simulink model "full_controlled_rect"  (R2017a)
settings: Solver=FixedStepAuto  StartTime=0.0  StopTime=15  RelTol=1e-3  EnableMultiTasking=on
libraries: powerlib x9, powerlib_meascontrol x7
settings Model: Creator=Admin  LastModifiedBy=re
settings OptimizationCC: LifeSpan=inf
settings DebuggingCC: SFUnexpectedBacktrackingDiag=warning  SFNoUnconditionalDefaultTransitionDiag=warning  SFExecutionAtInitializationDiag=none
settings GRTTargetCC: TargetLangStandard=C89/C90 (ANSI)  GeneratePreprocessorConditionals=Disable all
settings ConfigComp: CovMetricSettings=dw  CovHtmlReporting=on  CovSaveCumulativeToWorkspaceVar=on  CovSaveSingleToWorkspaceVar=on  CovExternalEMLEnable=off

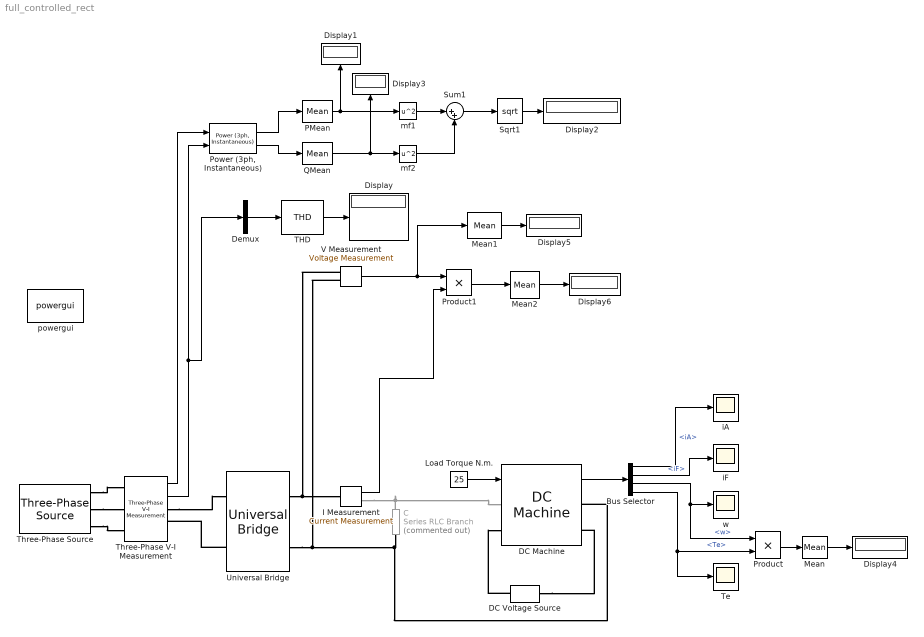
== system full_controlled_rect ==
  Bus Selector : BusSelector  OutputSignals=iA,iF,w,Te
  C : powerlib/Elements/Series RLC Branch  Commented=on  LConnTagsString=__new0  RConnTagsString=__new0  BranchType=RLC  Resistance=0  Inductance=0  SetiL0=off  InitialCurrent=0  Capacitance=100e-3  Setx0=off  InitialVoltage=0  Measurements=None
  DC Machine : powerlib/Machines/DC Machine  PresetModel=No  MechanicalLoad=Torque TL  FieldType=Wound  ShowDetailedParameters=on  MeasurementBus=on  RLa="[10  0.01]"  RLf="[300  156]"  Laf=2  MachineConstant=Torque constant (N.m/A)  Ke=1.8  Kt=1.8  J=1  Bm=0  Tf=0  w0=1  Ifinit=1  TsPowergui=0  TsBlock=-1
  DC Voltage Source : powerlib/Electrical Sources/DC Voltage Source  Amplitude=300  Measurements=None
  Demux : Demux  Outputs=1
  Display{,1..6} (7 alike) : Display
  I Measurement : powerlib/Measurements/Current Measurement  PhasorSimulation=off  OutputType=Complex  PSBequivalent=0
  Load Torque N.m. : Constant  Value=25
  Mean : powerlib_meascontrol/Measurements/Mean  Freq=60  Vinit=0  Ts=0
  Mean1 : powerlib_meascontrol/Measurements/Mean  Freq=60  Vinit=0  Ts=0
  Mean2 : powerlib_meascontrol/Measurements/Mean  Freq=60  Vinit=0  Ts=0
  PMean : powerlib_meascontrol/Measurements/Mean  Freq=60  Vinit=0  Ts=0
  "Power (3ph, Instantaneous)" : powerlib_meascontrol/Measurements/Power (3ph, Instantaneous)
      settings: SourceProductName=Simscape Power Systems
  Product : Product
  Product1 : Product
  QMean : powerlib_meascontrol/Measurements/Mean  Freq=60  Vinit=0  Ts=0
  Sqrt1 : Sqrt  SaturateOnIntegerOverflow=on
  Sum1 : Sum  Inputs=|++
  THD : powerlib_meascontrol/Measurements/THD  Freq=50  Ts=0
  Te : Scope
  Three-Phase V-I Measurement : powerlib/Measurements/Three-Phase V-I Measurement  VoltageMeasurement=phase-to-ground  SetLabelV=off  LabelV=Vabc  Vpu=off  VpuLL=off  CurrentMeasurement=yes  SetLabelI=off  LabelI=Iabc  Ipu=off  Pbase=100e6  Vbase=500e3  OutputType=Complex  PhasorSimulation=off  PSBequivalent=0
  Three-Phase Source : powerlib/Electrical Sources/Three-Phase Source  InternalConnection=Yg  VoltagePhases=off  Voltage=400  PhaseAngle=0  Voltage_phases=[25e3 25e3 25e3]/sqrt(3)  PhaseAngles_phases=[0 -120 +120]  Frequency=50  NonIdealSource=on  SpecifyImpedance=off  Resistance=100e-3  Inductance=100e-6  ShortCircuitLevel=100e6  BaseVoltage=400  XRratio=7  BusType=swing  Pref=10e3  Qref=0  Prefabc=[10e3, 10e3, 10e3]  Qrefabc=[0, 0, 0]  Qmin=-inf  Qmax=inf
  Universal Bridge : powerlib/Power Electronics/Universal Bridge  Arms=2  SnubberResistance=1e5  SnubberCapacitance=inf  Device=Diodes  Ron=20e-3  Lon=0  ForwardVoltages="[  0  0  ]"  ForwardVoltage=0.8  GTOparameters=[ 10e-6 , 20e-6 ]  IGBTparameters=[ 1e-6 , 2e-6 ]  Measurements=None  Measurements_2=None  converterType=Rectifier
  V Measurement : powerlib/Measurements/Voltage Measurement  PhasorSimulation=off  OutputType=Complex  PSBequivalent=0
  iA : Scope
  iF : Scope
  mf1 : Math  Operator=square  SaturateOnIntegerOverflow=on
  mf2 : Math  Operator=square  SaturateOnIntegerOverflow=on
  powergui : powerlib/powergui  Priority=1  SimulationMode=Discrete  SampleTime=50e-6  frequency=60  Iterations=50  frequencyindice=0  Pbase=100e6  ErrMax=1e-4  UnitsV=kV  UnitsW=MW  buscounter=0  FunctionMessages=off  echomessages=off  EnableUseOfTLC=off  CurrentSourceSwitches=off  DisableSnubberDevices=off  DisableRonSwitches=off  DisableVfSwitches=off  DisplayEquations=off  SolverType=Tustin/Backward Euler (TBE)  Interpol=off  ExternalGateDelay=off  methode=off  Ts=100  x0status=blocks  SPID=off  SwTol=0  HookPort=off  RestoreLinks=warning  ResistiveCurrentMeasurement=off  Frange=[0:2:500]  Ylog=off  Xlog=on  ShowGrid=off  save=off  variable=ZData  structure=0  ZoomFFT=off  StartTime=0.0  cycles=1  DisplayStyle=1  fundamental=60  FreqAxis=off  MaxFrequency=1000  frequencyindicesteady=1  RmsSteady=1  display=off
  w : Scope
  wires:
  Load Torque N.m./1 -> DC Machine/1
  DC Machine/1 -> Bus Selector/1
  Bus Selector/1 -> iA/1  "<iA>"
  Bus Selector/2 -> iF/1  "<iF>"
  Bus Selector/3 -> w/1, Product/1  "<w>"
  Bus Selector/4 -> Te/1, Product/2  "<Te>"
  Three-Phase V-I Measurement/2 -> Demux/1, "Power (3ph, Instantaneous)"/2
  Demux/1 -> THD/1
  THD/1 -> Display/1
  Three-Phase V-I Measurement/1 -> "Power (3ph, Instantaneous)"/1
  "Power (3ph, Instantaneous)"/1 -> PMean/1
  "Power (3ph, Instantaneous)"/2 -> QMean/1
  PMean/1 -> mf1/1, Display1/1
  QMean/1 -> mf2/1, Display3/1
  mf1/1 -> Sum1/1
  mf2/1 -> Sum1/2
  Sum1/1 -> Sqrt1/1
  Sqrt1/1 -> Display2/1
  Product/1 -> Mean/1
  Mean/1 -> Display4/1
  V Measurement/1 -> Product1/1, Mean1/1
  Mean1/1 -> Display5/1
  I Measurement/1 -> Product1/2
  Product1/1 -> Mean2/1
  Mean2/1 -> Display6/1
  connections:
  DC Voltage Source/RConn1 -- DC Machine/LConn2
  DC Voltage Source/LConn1 -- DC Machine/RConn2
  C/LConn1 -- I Measurement/RConn1 -- DC Machine/LConn1
  Universal Bridge/RConn2 -- V Measurement/LConn2 -- C/RConn1 -- DC Machine/RConn1
  Three-Phase V-I Measurement/RConn1 -- Universal Bridge/LConn1
  Universal Bridge/LConn2 -- Three-Phase V-I Measurement/RConn2
  Three-Phase Source/RConn1 -- Three-Phase V-I Measurement/LConn1
  Three-Phase Source/RConn2 -- Three-Phase V-I Measurement/LConn2
  Three-Phase Source/RConn3 -- Three-Phase V-I Measurement/LConn3
  Universal Bridge/RConn1 -- V Measurement/LConn1 -- I Measurement/LConn1
